simulink model "simulinkteste"  (R2015a)
settings: Solver=ode45  StartTime=0.0  StopTime=inf  RelTol=1e-3
undefined symbols (not defined in the file or in its folder): a1, Ta
libraries: dsparch4 x1, commanabbnd3 x1, dspsrcs4 x1
settings Model: Creator=aluno  LastModifiedBy=aluno

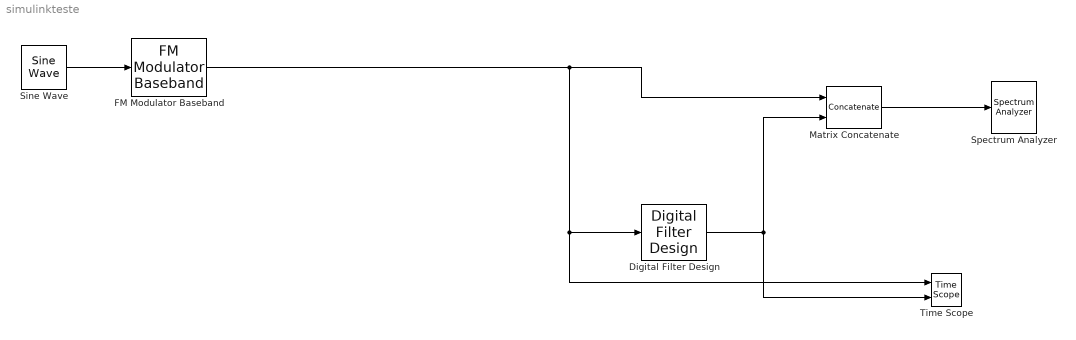
== system simulinkteste ==
  Digital Filter Design : dsparch4/Digital Filter Design  mwdsp_browser_bugfix_var=off
  FM Modulator Baseband : commanabbnd3/FM Modulator Baseband  FrequencyDeviation=100  SimulateUsing=Code generation
  Matrix Concatenate : Concatenate  Mode=Multidimensional array  ConcatenateDimension=2
  Sine Wave : dspsrcs4/Sine Wave  Amplitude=a1  Frequency=1  Phase=0  SampleMode=Discrete  OutComplex=Real  CompMethod=Differential  TableSize=Speed  SampleTime=Ta  SamplesPerFrame=spf  ResetState=Restart at time zero  dataType=double  wordLen=16  udDataType=sfix(16)  fracBitsMode=Best precision  numFracBits=15  OutDataTypeStr=double  LastOutDataTypeStr=double
  Spectrum Analyzer : SpectrumAnalyzer
  Time Scope : TimeScope  DefaultConfigurationName=spbscopes.TimeScopeBlockCfg  NumInputPorts=2
  wires:
  FM Modulator Baseband/1 -> Digital Filter Design/1, Time Scope/1, Matrix Concatenate/1
  Matrix Concatenate/1 -> Spectrum Analyzer/1
  Digital Filter Design/1 -> Time Scope/2, Matrix Concatenate/2
  Sine Wave/1 -> FM Modulator Baseband/1
